simulink model "VisionModel"  (Simulink 7.6)
settings: Solver=FixedStepDiscrete  StartTime=0.0  StopTime=0  RelTol=1e-3
settings Model: Creator=Administrator  LastModifiedBy=auvt
settings OptimizationCC: OptimizeModelRefInitCode=on
settings RTWCC: SystemTargetFile=ert.tlc  GenCodeOnly=on  TemplateMakefile=ert_default_tmf  PostCodeGenCommand=packNGo(buildInfo, {'packType' 'flat'})  Description=Real-Time Workshop Embedded Coder  GenerateReport=on  ProcessScript=ert_make_rtw_hook  IncludeHyperlinkInReport=on  LaunchReport=on  TargetLang=C++
settings CodeAppCC: IgnoreCustomStorageClasses=off
settings ERTTargetCC: MultiwordLength=2048  GenerateSampleERTMain=on  ERTCustomFileTemplate=example_file_process.tlc  ConvertIfToSwitch=off

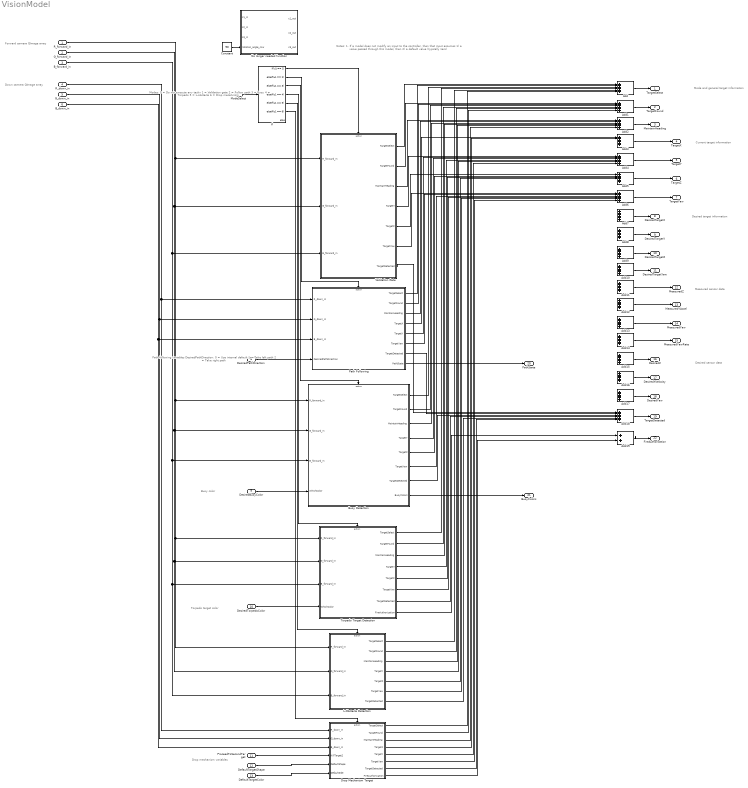
== system VisionModel ==
  note: Current target information
  note: Desired target information
  note: Measured sensor data
  note: Mode and general target information
  note: Desired sensor data
  note: Forward camera QImage array
  note: Modes:
      | 0 = Do not execute any tasks
      | 1 = Validation gate
      | 2 = Follow path
      | 3 = Buoy
      | 4 = Torpedo
      | 5 = L-obstacle
      | 6 = Drop mecahnism
  note: Path-following variables
      | DesiredPathDirection:
      | 0 = Use internal default
      | 1 = Take left path
      | 2 = Take right path
  note: Buoy color
  note: Torpedo target color
  note: Drop mechanism variables
  note: Down camera QImage array
  note: Notes:
      | 1. If a model does not modify an input to the controller,
      | then that input assumes 1) a value passed through this
      | model, then 2) a default value (typically zero)
  R_forward_in : Inport  PortDimensions=[160 120]
  G_forward_in : Inport  Port=2  PortDimensions=[160 120]
  B_forward_in : Inport  Port=3  PortDimensions=[160 120]
  R_down_in : Inport  Port=4  PortDimensions=[120 160]
  G_down_in : Inport  Port=5  PortDimensions=[120 160]
  B_down_in : Inport  Port=6  PortDimensions=[120 160]
  ModeSelect : Inport  Port=7
  DesiredPathDirection : Inport  Port=8
  DesiredBuoyColor : Inport  Port=9
  DesiredTorpedoColor : Inport  Port=10
  ProceedToSecondTarget : Inport  Port=11
  DefaultTargetShape : Inport  Port=12
  DefaultTargetColor : Inport  Port=13
  Add{,1..18} (19 alike) : Sum  Inputs=++++++
  Add19 : Sum
  Buoy Detection : Subsystem  TreatAsAtomicUnit=on
  Constant : Constant  Value=90  SampleTime=-1
  Drop Mechanism Target : Subsystem  TreatAsAtomicUnit=on
  If : If  IfExpression=u1 == 1  ElseIfExpressions=u1 == 2, u1 == 3, u1 == 4, u1 == 5, u1 == 6
  L-Obstacle Detection : Subsystem  TreatAsAtomicUnit=on
  No longer needed function : Stateflow chart  TreatAsAtomicUnit=on
  Path Following : Subsystem  TreatAsAtomicUnit=on
  Torpedo Target Detection : Subsystem  TreatAsAtomicUnit=on
  Validation Gate : Subsystem  TreatAsAtomicUnit=on
  TargetSelect : Outport  OutDataTypeStr=double
  TargetFound : Outport  Port=2  OutDataTypeStr=double
  MaintainHeading : Outport  Port=3  OutDataTypeStr=double
  TargetX : Outport  Port=4  OutDataTypeStr=double
  TargetY : Outport  Port=5  OutDataTypeStr=double
  TargetZ : Outport  Port=6  OutDataTypeStr=double
  TargetYaw : Outport  Port=7  OutDataTypeStr=double
  DesiredTargetX : Outport  Port=8  OutDataTypeStr=double
  DesiredTargetY : Outport  Port=9  OutDataTypeStr=double
  DesiredTargetZ : Outport  Port=10  OutDataTypeStr=double
  DesiredTargetYaw : Outport  Port=11  OutDataTypeStr=double
  MeasuredZ : Outport  Port=12  OutDataTypeStr=double
  MeasuredYAccel : Outport  Port=13  OutDataTypeStr=double
  MeasuredYaw : Outport  Port=14  OutDataTypeStr=double
  MeasuredYawRate : Outport  Port=15  OutDataTypeStr=double
  DesiredZ : Outport  Port=16  OutDataTypeStr=double
  DesiredXVelocity : Outport  Port=17  OutDataTypeStr=double
  DesiredYaw : Outport  Port=18  OutDataTypeStr=double
  TargetDetected : Outport  Port=19  OutDataTypeStr=double
  PathState : Outport  Port=20  OutDataTypeStr=double
  BuoyColors : Outport  Port=21  OutDataTypeStr=double
  FireAuthorization : Outport  Port=22  OutDataTypeStr=double
  wires:
  ModeSelect/1 -> If/1
  If/2 -> Path Following/Action
  If/3 -> Buoy Detection/Action
  If/1 -> Validation Gate/Action
  If/4 -> Torpedo Target Detection/Action
  If/5 -> L-Obstacle Detection/Action
  If/6 -> Drop Mechanism Target/Action
  DesiredBuoyColor/1 -> Buoy Detection/4(WhichColor)
  R_down_in/1 -> Path Following/1(R_down_in), Drop Mechanism Target/1(R_down_in)
  G_down_in/1 -> Path Following/2(G_down_in), Drop Mechanism Target/2(G_down_in)
  B_down_in/1 -> Path Following/3(B_down_in), Drop Mechanism Target/3(B_down_in)
  Add3/1 -> TargetX/1
  Add4/1 -> TargetY/1
  Add5/1 -> TargetZ/1
  Add6/1 -> TargetYaw/1
  Add7/1 -> DesiredTargetX/1
  Add8/1 -> DesiredTargetY/1
  Add9/1 -> DesiredTargetZ/1
  Add10/1 -> DesiredTargetYaw/1
  Add11/1 -> MeasuredZ/1
  Add12/1 -> MeasuredYAccel/1
  Add13/1 -> MeasuredYaw/1
  Add14/1 -> MeasuredYawRate/1
  Add15/1 -> DesiredZ/1
  Add16/1 -> DesiredXVelocity/1
  Add17/1 -> DesiredYaw/1
  Constant/1 -> No longer needed function/4(rotation_angle_ccw)
  R_forward_in/1 -> Validation Gate/1(R_forward_in), Buoy Detection/1(R_forward_in), Torpedo Target Detection/1(R_forward_in), L-Obstacle Detection/1(R_forward_in)
  G_forward_in/1 -> Validation Gate/2(G_forward_in), Buoy Detection/2(G_forward_in), Torpedo Target Detection/2(G_forward_in), L-Obstacle Detection/2(G_forward_in)
  B_forward_in/1 -> Validation Gate/3(B_forward_in), Buoy Detection/3(B_forward_in), Torpedo Target Detection/3(B_forward_in), L-Obstacle Detection/3(B_forward_in)
  Add18/1 -> TargetDetected/1
  Buoy Detection/8(BuoyColors) -> BuoyColors/1
  Add1/1 -> TargetFound/1
  Add/1 -> TargetSelect/1
  Add2/1 -> MaintainHeading/1
  Validation Gate/1(TargetSelect) -> Add/1
  Validation Gate/2(TargetFound) -> Add1/1
  Validation Gate/3(MaintainHeading) -> Add2/1
  Validation Gate/4(TargetY) -> Add4/1
  Validation Gate/5(TargetZ) -> Add5/1
  Validation Gate/6(TargetYaw) -> Add6/1
  Validation Gate/7(TargetDetected) -> Add18/1
  Path Following/1(TargetSelect) -> Add/2
  Path Following/2(TargetFound) -> Add1/2
  Path Following/3(MaintainHeading) -> Add2/2
  Path Following/4(TargetX) -> Add3/1
  Path Following/5(TargetY) -> Add4/2
  Path Following/6(TargetYaw) -> Add6/2
  Path Following/7(TargetDetected) -> Add18/2
  Path Following/8(PathState) -> PathState/1
  Buoy Detection/1(TargetSelect) -> Add/3
  Buoy Detection/2(TargetFound) -> Add1/3
  Buoy Detection/3(MaintainHeading) -> Add2/3
  Buoy Detection/4(TargetY) -> Add4/3
  Buoy Detection/5(TargetZ) -> Add5/2
  Buoy Detection/6(TargetYaw) -> Add6/3
  Buoy Detection/7(TargetDetected) -> Add18/3
  Torpedo Target Detection/1(TargetSelect) -> Add/4
  Torpedo Target Detection/2(TargetFound) -> Add1/4
  Torpedo Target Detection/3(MaintainHeading) -> Add2/4
  Torpedo Target Detection/4(TargetY) -> Add4/4
  Torpedo Target Detection/5(TargetZ) -> Add5/3
  Torpedo Target Detection/6(TargetYaw) -> Add6/4
  Torpedo Target Detection/7(TargetDetected) -> Add18/4
  L-Obstacle Detection/1(TargetSelect) -> Add/5
  L-Obstacle Detection/2(TargetFound) -> Add1/5
  L-Obstacle Detection/3(MaintainHeading) -> Add2/5
  L-Obstacle Detection/5(TargetZ) -> Add5/4
  L-Obstacle Detection/6(TargetYaw) -> Add6/5
  L-Obstacle Detection/4(TargetY) -> Add4/5
  L-Obstacle Detection/7(TargetDetected) -> Add18/5
  Drop Mechanism Target/1(TargetSelect) -> Add/6
  Drop Mechanism Target/2(TargetFound) -> Add1/6
  Drop Mechanism Target/3(MaintainHeading) -> Add2/6
  Drop Mechanism Target/4(TargetX) -> Add3/2
  Drop Mechanism Target/5(TargetY) -> Add4/6
  Drop Mechanism Target/6(TargetYaw) -> Add6/6
  Drop Mechanism Target/7(TargetDetected) -> Add18/6
  Drop Mechanism Target/8(FireAuthorization) -> Add19/2
  Add19/1 -> FireAuthorization/1
  Torpedo Target Detection/8(FireAuthorization) -> Add19/1
  DesiredPathDirection/1 -> Path Following/4(DesiredPathDirection)
  DesiredTorpedoColor/1 -> Torpedo Target Detection/4(WhichColor)
  ProceedToSecondTarget/1 -> Drop Mechanism Target/4(KillTarget2)
  DefaultTargetShape/1 -> Drop Mechanism Target/5(DefaultShape)
  DefaultTargetColor/1 -> Drop Mechanism Target/6(DefaultSide)

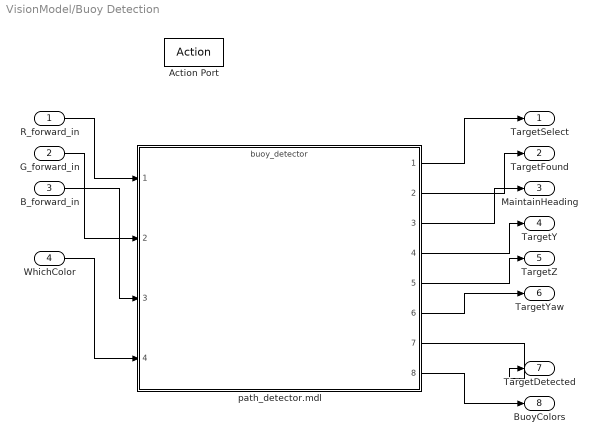
== system VisionModel/Buoy Detection ==
  R_forward_in : Inport  PortDimensions=[160 120]
  G_forward_in : Inport  Port=2  PortDimensions=[160 120]
  B_forward_in : Inport  Port=3  PortDimensions=[160 120]
  WhichColor : Inport  Port=4
  Action Port : ActionPort  ActionType=elseif
  path_detector.mdl : ModelReference  ModelNameDialog=buoy_detector  SimulationMode=Accelerator  ModelReferenceVersion=1.713  CopyOfModelName=buoy_detector
  TargetSelect : Outport  OutDataTypeStr=double
  TargetFound : Outport  Port=2  OutDataTypeStr=double
  MaintainHeading : Outport  Port=3  OutDataTypeStr=double
  TargetY : Outport  Port=4  OutDataTypeStr=double
  TargetZ : Outport  Port=5  OutDataTypeStr=double
  TargetYaw : Outport  Port=6  OutDataTypeStr=double
  TargetDetected : Outport  Port=7  OutDataTypeStr=double
  BuoyColors : Outport  Port=8  OutDataTypeStr=double
  wires:
  path_detector.mdl/1 -> TargetSelect/1
  path_detector.mdl/2 -> TargetFound/1
  path_detector.mdl/3 -> MaintainHeading/1
  path_detector.mdl/4 -> TargetY/1
  path_detector.mdl/5 -> TargetZ/1
  path_detector.mdl/6 -> TargetYaw/1
  path_detector.mdl/7 -> TargetDetected/1
  path_detector.mdl/8 -> BuoyColors/1
  R_forward_in/1 -> path_detector.mdl/1
  G_forward_in/1 -> path_detector.mdl/2
  B_forward_in/1 -> path_detector.mdl/3
  WhichColor/1 -> path_detector.mdl/4

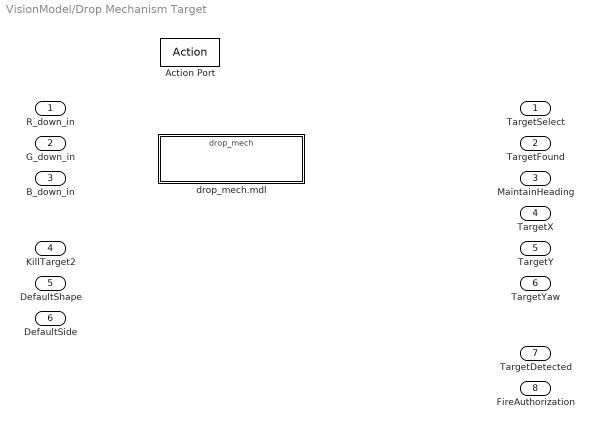
== system VisionModel/Drop Mechanism Target ==
  R_down_in : Inport
  G_down_in : Inport  Port=2
  B_down_in : Inport  Port=3
  KillTarget2 : Inport  Port=4
  DefaultShape : Inport  Port=5
  DefaultSide : Inport  Port=6
  Action Port : ActionPort  ActionType=elseif
  drop_mech.mdl : ModelReference  ModelNameDialog=drop_mech  SimulationMode=Accelerator  ModelReferenceVersion=1.6  CopyOfModelName=drop_mech
  TargetSelect : Outport  OutDataTypeStr=double
  TargetFound : Outport  Port=2  OutDataTypeStr=double
  MaintainHeading : Outport  Port=3  OutDataTypeStr=double
  TargetX : Outport  Port=4  OutDataTypeStr=double
  TargetY : Outport  Port=5  OutDataTypeStr=double
  TargetYaw : Outport  Port=6  OutDataTypeStr=double
  TargetDetected : Outport  Port=7  OutDataTypeStr=double
  FireAuthorization : Outport  Port=8  OutDataTypeStr=double

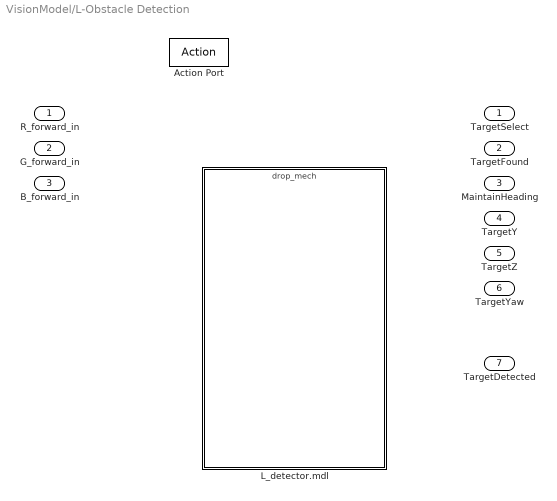
== system VisionModel/L-Obstacle Detection ==
  R_forward_in : Inport
  G_forward_in : Inport  Port=2
  B_forward_in : Inport  Port=3
  Action Port : ActionPort  ActionType=elseif
  L_detector.mdl : ModelReference  ModelNameDialog=drop_mech  SimulationMode=Accelerator  ModelReferenceVersion=1.6  CopyOfModelName=drop_mech
  TargetSelect : Outport  OutDataTypeStr=double
  TargetFound : Outport  Port=2  OutDataTypeStr=double
  MaintainHeading : Outport  Port=3  OutDataTypeStr=double
  TargetY : Outport  Port=4  OutDataTypeStr=double
  TargetZ : Outport  Port=5  OutDataTypeStr=double
  TargetYaw : Outport  Port=6  OutDataTypeStr=double
  TargetDetected : Outport  Port=7  OutDataTypeStr=double

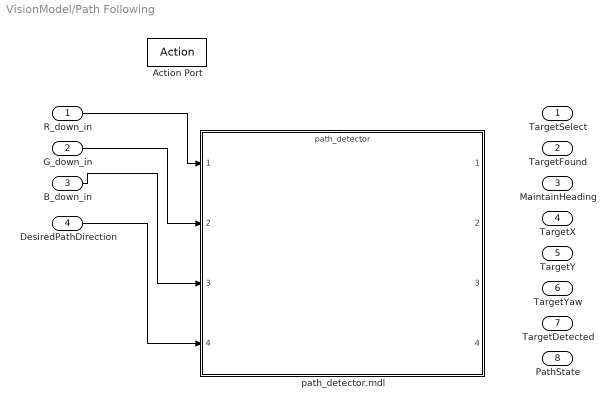
== system VisionModel/Path Following ==
  R_down_in : Inport
  G_down_in : Inport  Port=2
  B_down_in : Inport  Port=3
  DesiredPathDirection : Inport  Port=4
  Action Port : ActionPort  ActionType=elseif
  path_detector.mdl : ModelReference  ModelNameDialog=path_detector  SimulationMode=Accelerator  ModelReferenceVersion=1.220  CopyOfModelName=path_detector
  TargetSelect : Outport  OutDataTypeStr=double
  TargetFound : Outport  Port=2  OutDataTypeStr=double
  MaintainHeading : Outport  Port=3  OutDataTypeStr=double
  TargetX : Outport  Port=4  OutDataTypeStr=double
  TargetY : Outport  Port=5  OutDataTypeStr=double
  TargetYaw : Outport  Port=6  OutDataTypeStr=double
  TargetDetected : Outport  Port=7  OutDataTypeStr=double
  PathState : Outport  Port=8  OutDataTypeStr=double
  wires:
  R_down_in/1 -> path_detector.mdl/1
  G_down_in/1 -> path_detector.mdl/2
  B_down_in/1 -> path_detector.mdl/3
  DesiredPathDirection/1 -> path_detector.mdl/4

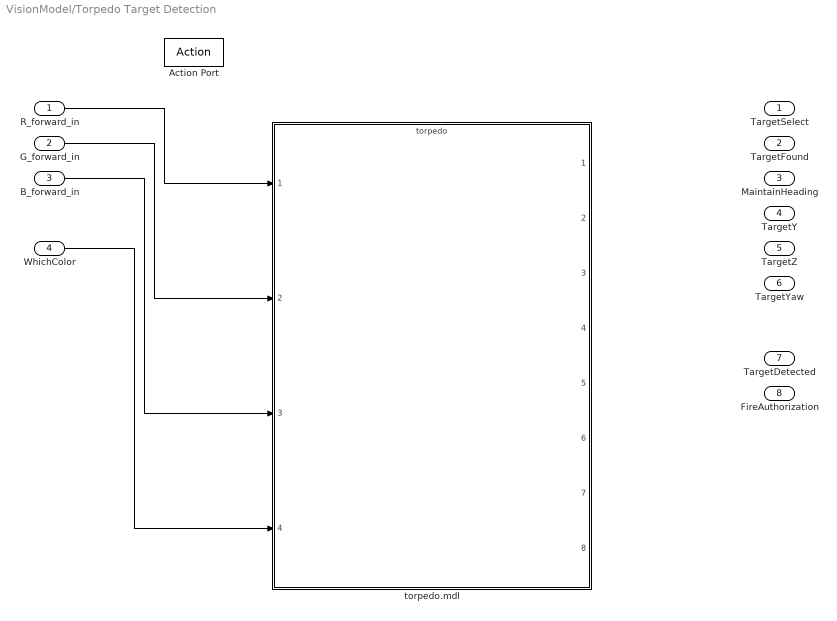
== system VisionModel/Torpedo Target Detection ==
  R_forward_in : Inport
  G_forward_in : Inport  Port=2
  B_forward_in : Inport  Port=3
  WhichColor : Inport  Port=4
  Action Port : ActionPort  ActionType=elseif
  torpedo.mdl : ModelReference  ModelNameDialog=torpedo  SimulationMode=Accelerator  ModelReferenceVersion=1.62  CopyOfModelName=torpedo
  TargetSelect : Outport  OutDataTypeStr=double
  TargetFound : Outport  Port=2  OutDataTypeStr=double
  MaintainHeading : Outport  Port=3  OutDataTypeStr=double
  TargetY : Outport  Port=4  OutDataTypeStr=double
  TargetZ : Outport  Port=5  OutDataTypeStr=double
  TargetYaw : Outport  Port=6  OutDataTypeStr=double
  TargetDetected : Outport  Port=7  OutDataTypeStr=double
  FireAuthorization : Outport  Port=8  OutDataTypeStr=double
  wires:
  R_forward_in/1 -> torpedo.mdl/1
  G_forward_in/1 -> torpedo.mdl/2
  B_forward_in/1 -> torpedo.mdl/3
  WhichColor/1 -> torpedo.mdl/4

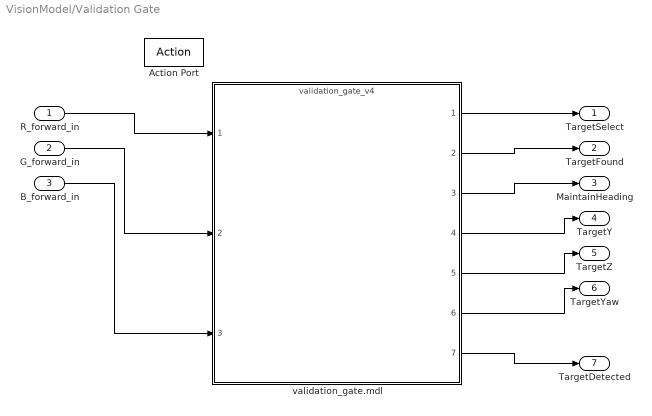
== system VisionModel/Validation Gate ==
  R_forward_in : Inport
  G_forward_in : Inport  Port=2
  B_forward_in : Inport  Port=3
  Action Port : ActionPort  ActionType=then
  validation_gate.mdl : ModelReference  ModelNameDialog=validation_gate_v4  SimulationMode=Accelerator  ModelReferenceVersion=1.1120  CopyOfModelName=validation_gate_v4
  TargetSelect : Outport  OutDataTypeStr=double
  TargetFound : Outport  Port=2  OutDataTypeStr=double
  MaintainHeading : Outport  Port=3  OutDataTypeStr=double
  TargetY : Outport  Port=4  OutDataTypeStr=double
  TargetZ : Outport  Port=5  OutDataTypeStr=double
  TargetYaw : Outport  Port=6  OutDataTypeStr=double
  TargetDetected : Outport  Port=7  OutDataTypeStr=double
  wires:
  R_forward_in/1 -> validation_gate.mdl/1
  G_forward_in/1 -> validation_gate.mdl/2
  B_forward_in/1 -> validation_gate.mdl/3
  validation_gate.mdl/7 -> TargetDetected/1
  validation_gate.mdl/1 -> TargetSelect/1
  validation_gate.mdl/2 -> TargetFound/1
  validation_gate.mdl/3 -> MaintainHeading/1
  validation_gate.mdl/4 -> TargetY/1
  validation_gate.mdl/5 -> TargetZ/1
  validation_gate.mdl/6 -> TargetYaw/1

== matlab function No longer needed function ==
  data: c1_in input double; c2_in input double; c3_in input double; c1_out output double; rotation_angle_ccw input double; c2_out output double; c3_out output double
function [c1_out, c2_out, c3_out] = rotateImage(c1_in, c2_in, c3_in, rotation_angle_ccw)
%#eml

% This function rotates an image in 90 degree increments
%
% Input
%   c1_in = input image component 1 data
%                   Note: Must be a 2-D (single color component) or 3-D
%                     (RGB or similar) array; first two dimensions
%                     specify image height and width, respectively
%   c2_in = input image component 2 data
%   c3_in = input image component 3 data
%
% Output
%   c1_out = output image component 1 data
%   c1_out = output image component 2 data
%   c1_out = output image component 3 data

% Determine loop indices
[m, n, depth] = size(c1_in);


% Initialize output
c1_out = double(zeros([120 160]));
c2_out = double(zeros([120 160]));
c3_out = double(zeros([120 160]));


% Loop
for i = 1:m
    for j = 1:n
        if(rotation_angle_ccw == 0)
            c1_out(i,j,:) = c1_in(i,j,:);
            c2_out(i,j,:) = c2_in(i,j,:);
            c3_out(i,j,:) = c3_in(i,j,:);
        elseif(rotation_angle_ccw == 90)
            c1_out(n-j+1,i,:) = c1_in(i,j,:);
            c2_out(n-j+1,i,:) = c2_in(i,j,:);
            c3_out(n-j+1,i,:) = c3_in(i,j,:);
%        elseif(rotation_angle_ccw == 180)
%            image_out(m-i+1,n-j+1) = image_in(i,j,:);
%        elseif(rotation_angle_ccw == 270)
%            image_out(j,m-i+1) = image_in(i,j,:);
        end
    end
end


return
